simulink model "PMSM_PLL_MTPA"  (R2018b)
settings: Solver=VariableStepAuto  StartTime=0.0  StopTime=20  FixedStep=Ts  RelTol=1e-4  EnableMultiTasking=on
InitFcn:
  | Ts = 1e-4;
  | 
  | Rs = 0.8975;
  | Ld = 15e-3;
  | Lq = 19e-3;
  | Pn = 3;
  | flux = 0.1764;
  | 
  | Kp_PLL = 150;
  | Ki_PLL = 100;
undefined symbols (not defined in the file or in its folder): DiscIntNeverNeededParam
libraries: powerlib x5, powerlib_extras x2, simulink x2
settings Model: Creator=SUN  LastModifiedBy=liangjin
settings SolverCC: ZeroCrossControl=DisableAll
settings DataIOCC: LimitDataPoints=on  SaveFormat=Array
settings OptimizationCC: ExpressionDepthLimit=2147483647  InitFltsAndDblsToZero=on  LifeSpan=inf
settings DebuggingCC: UnderspecifiedInitializationDetection=Classic  MergeDetectMultiDrivingBlocksExec=none  SolverPrmCheckMsg=warning  FcnCallInpInsideContextMsg=warning  StateNameClashWarn=warning  SFUnexpectedBacktrackingDiag=warning  SFNoUnconditionalDefaultTransitionDiag=warning  SFExecutionAtInitializationDiag=none
settings HardwareCC: ProdBitPerPointer=32  ProdBitPerSizeT=32  ProdBitPerPtrDiffT=32  ProdLargestAtomicFloat=None  ProdIntDivRoundTo=Undefined  ProdEndianess=Unspecified  ProdWordSize=32  ProdHWDeviceType=32-bit Generic
settings ModelReferenceCC: PropagateSignalLabelsOutOfModel=off
settings SFSimCC: SimUseLocalCustomCode=off
settings RTWCC: RTWUseLocalCustomCode=off
settings CodeAppCC: StateflowObjectComments=on
settings GRTTargetCC: TargetLangStandard=C89/C90 (ANSI)  GeneratePreprocessorConditionals=Disable all  CombineOutputUpdateFcns=off  GRTInterface=on
settings ConfigComp: CovMetricSettings=dw  CovHtmlReporting=on  CovSaveCumulativeToWorkspaceVar=on  CovSaveSingleToWorkspaceVar=on  CovExternalEMLEnable=off  CovSFcnEnable=off
settings SimscapeCC: SimscapeNormalizeSystem=off

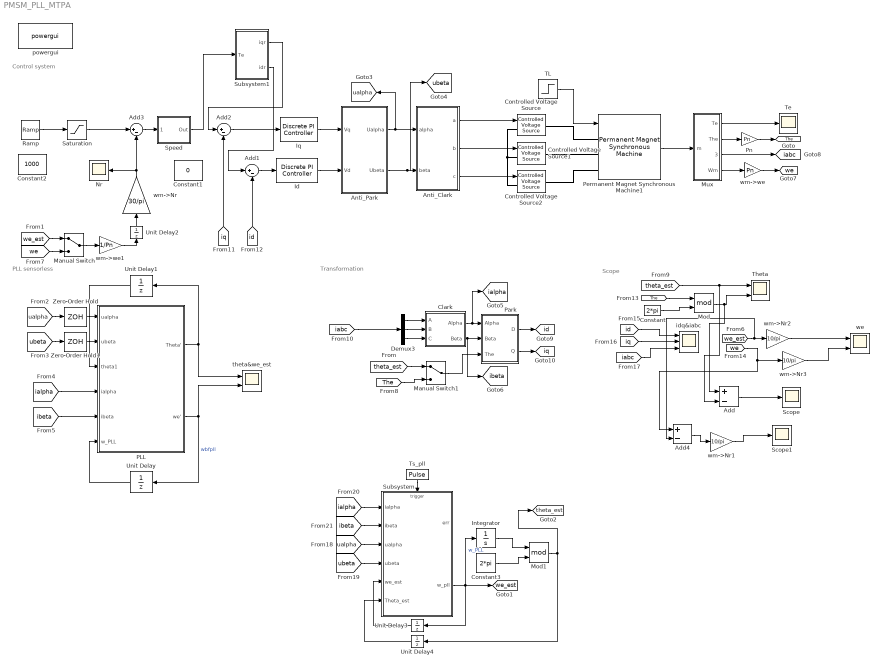
== system PMSM_PLL_MTPA ==
  note: Scope
  note: Control system
  note: Transformation
  note: PLL sensorless
  Add : Sum  Inputs=+-
  Add1 : Sum  Inputs=|+-
  Add2 : Sum  Inputs=|+-
  Add3 : Sum  Inputs=|+-
  Add4 : Sum  Inputs=+-
  Anti_Clark : Subsystem
  Anti_Park : Subsystem
  Clark : Subsystem
  Constant : Constant  Value=2*pi
  Constant1 : Constant  Value=0
  Constant2 : Constant  Value=1000
  Constant3 : Constant  Value=2*pi
  Controlled Voltage Source : powerlib/Electrical Sources/Controlled Voltage Source  Initialize=on  Source_Type=AC  Amplitude=0  Phase=0  Frequency=0  Measurements=None
      settings: SourceProductName=Simscape Electrical
  Controlled Voltage Source1 : powerlib/Electrical Sources/Controlled Voltage Source  Initialize=on  Source_Type=AC  Amplitude=0  Phase=0  Frequency=0  Measurements=None
      settings: SourceProductName=Simscape Electrical
  Controlled Voltage Source2 : powerlib/Electrical Sources/Controlled Voltage Source  Initialize=on  Source_Type=AC  Amplitude=0  Phase=0  Frequency=0  Measurements=None
      settings: SourceProductName=Simscape Electrical
  Demux3 : Demux  Outputs=3
  Id : powerlib_extras/Discrete  Control Blocks/Discrete PI Controller  Kp=Ld*376  Ki=Rs*376  Par_Limits=[311*0.9*sqrt(1/3) -311*0.9*sqrt(1/3)]  Init=0  Ts=Ts
  Integrator : Integrator
  Iq : powerlib_extras/Discrete  Control Blocks/Discrete PI Controller  Kp=Lq*376  Ki=Rs*376  Par_Limits=[311*0.9*sqrt(1/3) -311*0.9*sqrt(1/3)]  Init=0  Ts=Ts
  Manual Switch : ManualSwitch
  Manual Switch1 : ManualSwitch
  Mod : Math  Operator=mod  SaturateOnIntegerOverflow=on
  Mod1 : Math  Operator=mod  SaturateOnIntegerOverflow=on
  Mux : Subsystem
  Nr : Scope
  PLL : Subsystem
  Park : Subsystem
  Permanent Magnet Synchronous Machine1 : powerlib/Machines/Permanent Magnet Synchronous Machine  NbPhases=3  FluxDistribution=Sinusoidal  RotorType=Salient-pole  MechanicalLoad=Torque Tm  PresetModel=No  ShowDetailedParameters=on  MeasurementBus=off  Resistance=0.8975  Inductance=8.5e-3  dqInductances=[1.3*15e-3,1.3*19e-3]  La=0.000835  MachineConstant=Flux linkage established by magnets (V.s)  Flux=0.1764  VoltageCst=95.9863  TorqueCst=0.7938  Flat=120  Mechanical=[0.000311 0.0000001 3]  PolePairs=3  InitialConditions=[0,0, 0,0]  InitialConditions5ph=[0 0 0 0 0 0]  TsPowergui=0  TsBlock=Ts  RefAngle=Aligned with phase A axis (original Park)
  Pn : Gain  Gain=Pn
  Ramp : simulink/Sources/Ramp  slope=250  start=0  InitialOutput=0
  Saturation : Saturate  UpperLimit=1000  LowerLimit=-1000
  Scope : Scope
  Scope1 : Scope
  Speed : Subsystem  AncestorBlock=|  DialogController=POWERSYS.PowerSysDialog  mask(Discrete PI Controller){Kpw=0.01, Kiw=0.01*50, Ba=0, Par_Limits=[30 -30], Init=0, Ts=Ts*10}
      | powerlib_extras/Discrete 
      | Control Blocks/Discrete
      | PI Controller
      mask prompts: Kpw "Proportional gain (Kp):"; Kiw "Integral gain (Ki):"; Ba "feedback gain (Ba)"; Par_Limits "Output limits: [ Upper   Lower ]"; Init "Output initial value:"; Ts "Sample time:"
      mask help: This block implements a discrete PI controller.
      mask init:
      | UpperLimit=Par_Limits(1);
      | LowerLimit=Par_Limits(2);
      | power_initmask();
      mask Help: This block is part of a subset of blocks in the Extras library that does not have documentation associated with it, other than the block mask description.
      mask Display: disp('PI');
  Subsystem : Subsystem
  Subsystem1 : Subsystem
  TL : Step  Time=5  After=3  SampleTime=Ts
  Te : Scope
  Theta : Scope  NumInputPorts=2
  Ts_pll : DiscretePulseGenerator  PulseType=Time based  Period=Ts  PulseWidth=50
  Unit Delay{,1,3..4} (4 alike) : UnitDelay  SampleTime=Ts
  Unit Delay2 : UnitDelay  SampleTime=-1
  Zero-Order Hold : ZeroOrderHold  SampleTime=Ts
  Zero-Order Hold1 : ZeroOrderHold  SampleTime=Ts
  idq&iabc : Scope  NumInputPorts=3
  powergui : powerlib/powergui  SimulationMode=Continuous  SampleTime=Ts*10  frequency=60  Iterations=50  frequencyindice=0  Pbase=100e6  ErrMax=1e-4  UnitsV=kV  UnitsW=MW  buscounter=0  FunctionMessages=off  echomessages=off  EnableUseOfTLC=off  CurrentSourceSwitches=off  DisableSnubberDevices=off  DisableRonSwitches=off  DisableVfSwitches=off  DisplayEquations=off  SolverType=Tustin/Backward Euler (TBE)  Interpol=off  ExternalGateDelay=off  methode=off  Ts=100  x0status=blocks  SPID=off  SwTol=0  HookPort=off  RestoreLinks=warning  ResistiveCurrentMeasurement=off  Frange=[0:2:500]  Ylog=off  Xlog=on  ShowGrid=off  save=off  variable=ZData  structure=0  ZoomFFT=on  StartTime=0.0  cycles=1  DisplayStyle=1  fundamental=60  FreqAxis=off  MaxFrequency=1000  frequencyindicesteady=1  RmsSteady=1  display=off
  theta&we_est : Scope  NumInputPorts=2
  we : Scope  NumInputPorts=2
  wm->Nr : Gain  Gain=30/pi
  wm->Nr1 : Gain  Gain=10/pi
  wm->Nr2 : Gain  Gain=10/pi
  wm->Nr3 : Gain  Gain=10/pi
  wm->we : Gain  Gain=Pn
  wm->we1 : Gain  Gain=1/Pn
  tag scope: The=global, iabc=global, ialpha=global, ibeta=global, id=global, iq=global, theta_est=global, ualpha=global, ubeta=global, we=global, we_est=global
  wires:
  TL/1 -> Permanent Magnet Synchronous Machine1/1
  Permanent Magnet Synchronous Machine1/1 -> Mux/1(m)
  Add3/1 -> Speed/1(Error)
  Add1/1 -> Id/1
  wm->Nr/1 -> Add3/2, Nr/1
  Add2/1 -> Iq/1
  Mux/1(Te) -> Te/1
  Mux/2(The) -> Pn/1
  Pn/1 -> [The]
  Mux/4(Wm) -> wm->we/1
  Mux/3(Iabc) -> [iabc]
  Clark/1(Alpha) -> [ialpha], Park/1(Alpha)
  Demux3/1 -> Clark/1(A)
  Demux3/2 -> Clark/2(B)
  Demux3/3 -> Clark/3(C)
  Clark/2(Beta) -> Park/2(Beta), [ibeta]
  Iq/1 -> Anti_Park/1(Vq)
  Id/1 -> Anti_Park/2(Vd)
  Anti_Clark/1(a) -> Controlled Voltage Source/1
  Anti_Clark/2(b) -> Controlled Voltage Source1/1
  Anti_Clark/3(c) -> Controlled Voltage Source2/1
  PLL/2(we') -> Unit Delay/1, theta&we_est/2  "wbfpll"
  PLL/1(Theta') -> theta&we_est/1, Unit Delay1/1
  Constant/1 -> Mod/2
  Mod/1 -> Add/1, Theta/2
  Unit Delay/1 -> PLL/6(w_PLL)
  Unit Delay1/1 -> PLL/3(theta1)
  wm->we/1 -> [we]
  Ramp/1 -> Saturation/1
  [ialpha] -> PLL/4(ialpha)
  [ibeta] -> PLL/5(ibeta)
  Anti_Park/1(Ualpha) -> [ualpha], Anti_Clark/1(alpha)
  Anti_Park/2(Ubeta) -> [ubeta], Anti_Clark/2(beta)
  [we_est] -> Manual Switch/1
  [we] -> Manual Switch/2
  [theta_est] -> Manual Switch1/1
  Manual Switch1/1 -> Park/3(The)
  [The] -> Manual Switch1/2
  [ualpha] -> Zero-Order Hold/1
  Zero-Order Hold/1 -> PLL/1(ualpha)
  [ubeta] -> Zero-Order Hold1/1
  Zero-Order Hold1/1 -> PLL/2(ubeta)
  [theta_est] -> Add/2, Theta/1
  [iabc] -> Demux3/1
  Park/1(D) -> [id]
  Park/2(Q) -> [iq]
  [The] -> Mod/1
  [id] -> idq&iabc/1
  [iq] -> idq&iabc/2
  [iabc] -> idq&iabc/3
  [id] -> Add1/2
  [iq] -> Add2/2
  Manual Switch/1 -> wm->we1/1
  Add4/1 -> wm->Nr1/1
  wm->Nr1/1 -> Scope1/1
  [we] -> Add4/1, wm->Nr3/1
  [we_est] -> Add4/2, wm->Nr2/1
  Add/1 -> Scope/1
  wm->Nr2/1 -> we/1
  wm->Nr3/1 -> we/2
  wm->we1/1 -> Unit Delay2/1
  Unit Delay2/1 -> wm->Nr/1
  Saturation/1 -> Add3/1
  [ialpha] -> Subsystem/1(ialpha)
  [ibeta] -> Subsystem/2(ibeta)
  [ualpha] -> Subsystem/3(ualpha)
  [ubeta] -> Subsystem/4(ubeta)
  Ts_pll/1 -> Subsystem/Trigger
  Constant3/1 -> Mod1/2
  Integrator/1 -> Mod1/1
  Subsystem/2(w_pll) -> [we_est], Integrator/1, Unit Delay3/1  "w_PLL"
  Mod1/1 -> Unit Delay4/1, [theta_est]
  Unit Delay3/1 -> Subsystem/5(we_est)
  Unit Delay4/1 -> Subsystem/6(Theta_est)
  Speed/1(Out) -> Subsystem1/1(Te)
  Subsystem1/1(iqr) -> Add2/1
  Subsystem1/2(idr) -> Add1/1
  connections:
  Controlled Voltage Source/LConn1 -- Controlled Voltage Source2/LConn1 -- Controlled Voltage Source1/LConn1
  Controlled Voltage Source/RConn1 -- Permanent Magnet Synchronous Machine1/LConn1
  Controlled Voltage Source1/RConn1 -- Permanent Magnet Synchronous Machine1/LConn2
  Controlled Voltage Source2/RConn1 -- Permanent Magnet Synchronous Machine1/LConn3

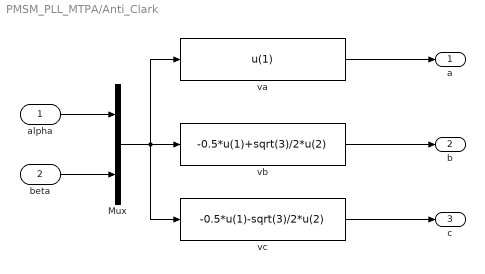
== system PMSM_PLL_MTPA/Anti_Clark ==
  alpha : Inport
  beta : Inport  Port=2
  Mux : Mux  Inputs=2
  va : Fcn  Expr=u(1)
  vb : Fcn  Expr=-0.5*u(1)+sqrt(3)/2*u(2)
  vc : Fcn  Expr=-0.5*u(1)-sqrt(3)/2*u(2)
  a : Outport
  b : Outport  Port=2
  c : Outport  Port=3
  wires:
  va/1 -> a/1
  beta/1 -> Mux/2
  alpha/1 -> Mux/1
  Mux/1 -> vc/1, vb/1, va/1
  vb/1 -> b/1
  vc/1 -> c/1

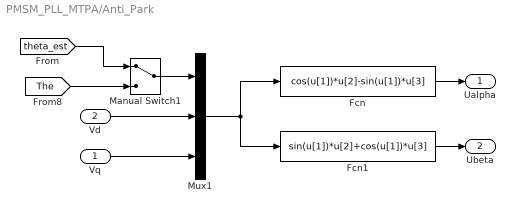
== system PMSM_PLL_MTPA/Anti_Park ==
  Vq : Inport
  Vd : Inport  Port=2
  Fcn : Fcn  Expr=cos(u[1])*u[2]-sin(u[1])*u[3]
  Fcn1 : Fcn  Expr=sin(u[1])*u[2]+cos(u[1])*u[3]
  Manual Switch1 : ManualSwitch
  Mux1 : Mux  Inputs=3
  Ualpha : Outport
  Ubeta : Outport  Port=2
  wires:
  Fcn1/1 -> Ubeta/1
  Fcn/1 -> Ualpha/1
  Mux1/1 -> Fcn/1, Fcn1/1
  Vd/1 -> Mux1/2
  Vq/1 -> Mux1/3
  Manual Switch1/1 -> Mux1/1
  [The] -> Manual Switch1/2
  [theta_est] -> Manual Switch1/1

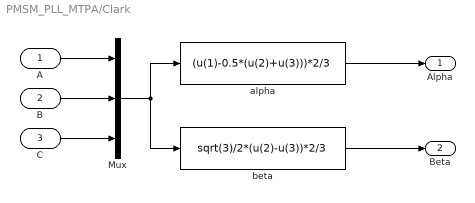
== system PMSM_PLL_MTPA/Clark ==
  A : Inport
  B : Inport  Port=2
  C : Inport  Port=3
  Mux : Mux  Inputs=3
  alpha : Fcn  Expr=(u(1)-0.5*(u(2)+u(3)))*2/3
  beta : Fcn  Expr=sqrt(3)/2*(u(2)-u(3))*2/3
  Alpha : Outport
  Beta : Outport  Port=2
  wires:
  alpha/1 -> Alpha/1
  B/1 -> Mux/2
  C/1 -> Mux/3
  A/1 -> Mux/1
  Mux/1 -> beta/1, alpha/1
  beta/1 -> Beta/1

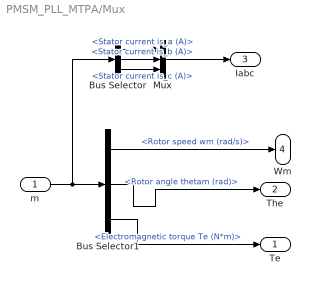
== system PMSM_PLL_MTPA/Mux ==
  m : Inport
  Bus Selector : BusSelector  OutputSignals=Stator current is_a (A),Stator current is_b (A),Stator current is_c (A)
  Bus Selector1 : BusSelector  OutputSignals=Rotor speed wm (rad/s),Rotor angle thetam (rad),Electromagnetic torque Te (N*m)
  Mux : Mux  Inputs=3
  Te : Outport
  The : Outport  Port=2
  Iabc : Outport  Port=3
  Wm : Outport  Port=4
  wires:
  Bus Selector1/1 -> Wm/1  "<Rotor speed wm (rad/s)>"
  Bus Selector1/2 -> The/1  "<Rotor angle thetam (rad)>"
  Bus Selector1/3 -> Te/1  "<Electromagnetic torque Te (N*m)>"
  m/1 -> Bus Selector/1, Bus Selector1/1
  Bus Selector/2 -> Mux/2  "<Stator current is_b (A)>"
  Bus Selector/3 -> Mux/3  "<Stator current is_c (A)>"
  Bus Selector/1 -> Mux/1  "<Stator current is_a (A)>"
  Mux/1 -> Iabc/1

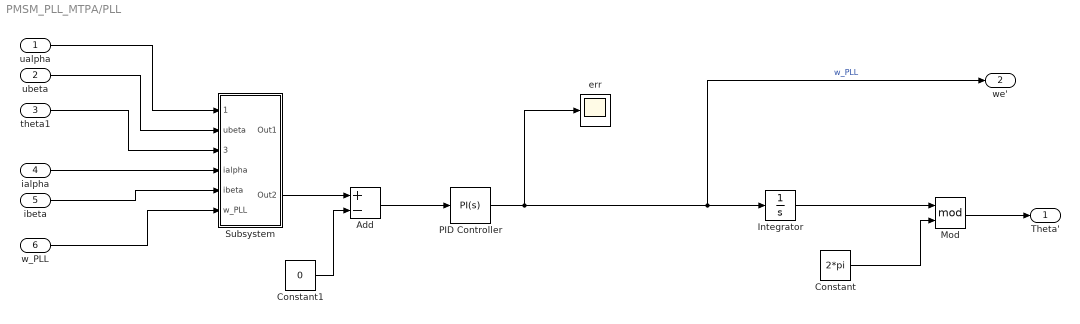
== system PMSM_PLL_MTPA/PLL ==
  ualpha : Inport
  ubeta : Inport  Port=2
  theta1 : Inport  Port=3
  ialpha : Inport  Port=4
  ibeta : Inport  Port=5
  w_PLL : Inport  Port=6
  Add : Sum  Inputs=+-
  Constant : Constant  Value=2*pi
  Constant1 : Constant  Value=0
  Integrator : Integrator
  Mod : Math  Operator=mod  SaturateOnIntegerOverflow=on
  PID Controller : simulink/Continuous/PID Controller  Controller=PI  Form=Parallel  TimeDomain=Continuous-time  SampleTime=-1  IntegratorMethod=Forward Euler  FilterMethod=Forward Euler  ControllerParametersSource=internal  P=Kp_PLL  I=Ki_PLL  D=0  UseFilter=on  N=100  TunerSelectOption=Transfer Function Based (PID Tuner App)  InitialConditionSource=internal  InitialConditionForIntegrator=0  InitialConditionForFilter=0  DifferentiatorICPrevScaledInput=0  ExternalReset=none  TrackingMode=off  Kt=1  LimitOutput=off  UpperSaturationLimit=inf  LowerSaturationLimit=-inf  LinearizeAsGain=on  AntiWindupMode=none  Kb=1  POutMin=[]  POutMax=[]  IOutMin=[]  IOutMax=[]  DOutMin=[]  DOutMax=[]  NOutMin=[]  NOutMax=[]  SumOutMin=[]  SumOutMax=[]  SaturationOutMin=[]  SaturationOutMax=[]  PParamMin=[]  PParamMax=[]  IParamMin=[]  IParamMax=[]  DParamMin=[]  DParamMax=[]  NParamMin=[]  NParamMax=[]  KbParamMin=[]  KbParamMax=[]  KtParamMin=[]  KtParamMax=[]  KbOutMin=[]  KbOutMax=[]  KtOutMin=[]  KtOutMax=[]  IntegratorOutMin=[]  IntegratorOutMax=[]  FilterOutMin=[]  FilterOutMax=[]  SumI1OutMin=[]  SumI1OutMax=[]  SumI2OutMin=[]  SumI2OutMax=[]  SumI3OutMin=[]  SumI3OutMax=[]  SumI4OutMin=[]  SumI4OutMax=[]  SumDOutMin=[]  SumDOutMax=[]  DifferentiatorOutMin=[]  DifferentiatorOutMax=[]  FilterDiffOutCoefMin=[]  FilterDiffOutCoefMax=[]  ReciprocalOutMin=[]  ReciprocalOutMax=[]  SumDenOutMin=[]  SumDenOutMax=[]  SumNumOutMin=[]  SumNumOutMax=[]  DivideOutMin=[]  DivideOutMax=[]  IntegratorContinuousStateAttributes=''  IntegratorStateMustResolveToSignalObject=off  IntegratorRTWStateStorageClass=Auto  FilterContinuousStateAttributes=''  FilterStateMustResolveToSignalObject=off  FilterRTWStateStorageClass=Auto  ParallelPVariant=InternalParameters  IdealPVariant=Disabled  IVariant=InternalParameters  DVariant=Disabled  IntegratorVariant=Continuous  SatVariant=Disabled  AWVariant=Passthrough  PCopyVariant=Disabled  TRVariant=Disabled  FdbkBlocksVariant=Forward  IdealPFdbkVariant=Disabled  SatFdbkVariant=Disabled  DerivativeFilterVariant=Disabled  NVariant=Disabled  NCopyVariant=Disabled_SignalSpec  FilterICVariant=Disabled  IntegratorICVariant=InternalICs  ExternalResetVariant=Disabled  TRSumVariant=Passthrough  SumFdbkVariant=Disabled  SumVariant=Sum_PI
  Subsystem : Subsystem
  err : Scope
  Theta' : Outport
  we' : Outport  Port=2
  wires:
  Constant/1 -> Mod/2
  Integrator/1 -> Mod/1
  Mod/1 -> Theta'/1
  ualpha/1 -> Subsystem/1(ualpha)
  ubeta/1 -> Subsystem/2(ubeta)
  ialpha/1 -> Subsystem/4(ialpha)
  ibeta/1 -> Subsystem/5(ibeta)
  theta1/1 -> Subsystem/3(theta1)
  w_PLL/1 -> Subsystem/6(w_PLL)
  Subsystem/2(Out2) -> Add/1
  Constant1/1 -> Add/2
  Add/1 -> PID Controller/1
  PID Controller/1 -> we'/1, Integrator/1, err/1  "w_PLL"

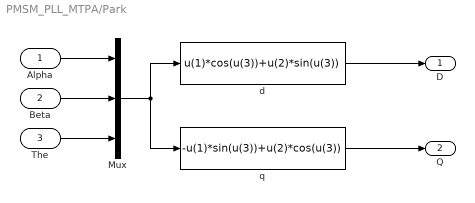
== system PMSM_PLL_MTPA/Park ==
  Alpha : Inport
  Beta : Inport  Port=2
  The : Inport  Port=3
  Mux : Mux  Inputs=3
  d : Fcn  Expr=u(1)*cos(u(3))+u(2)*sin(u(3))
  q : Fcn  Expr=-u(1)*sin(u(3))+u(2)*cos(u(3))
  D : Outport
  Q : Outport  Port=2
  wires:
  d/1 -> D/1
  Beta/1 -> Mux/2
  Alpha/1 -> Mux/1
  Mux/1 -> q/1, d/1
  q/1 -> Q/1
  The/1 -> Mux/3

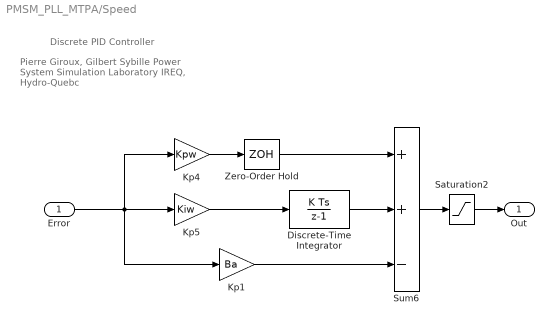
== system PMSM_PLL_MTPA/Speed ==
  note: Discrete PID Controller
  note: Pierre Giroux, Gilbert Sybille
      | Power System Simulation Laboratory
      | IREQ, Hydro-Quebc
  Error : Inport  SampleTime=Ts
  Discrete-Time Integrator : DiscreteIntegrator  InitialCondition=Init  SampleTime=Ts  LimitOutput=on  UpperSaturationLimit=UpperLimit  LowerSaturationLimit=LowerLimit  ICPrevOutput=DiscIntNeverNeededParam  ICPrevScaledInput=DiscIntNeverNeededParam
  Kp1 : Gain  Gain=Ba  SampleTime=Ts  SaturateOnIntegerOverflow=on  OutDataTypeStr=Inherit: Same as input  ParamDataTypeStr=Inherit: Same as input
  Kp4 : Gain  Gain=Kpw  SampleTime=Ts  SaturateOnIntegerOverflow=on  OutDataTypeStr=Inherit: Same as input  ParamDataTypeStr=Inherit: Same as input
  Kp5 : Gain  Gain=Kiw  SampleTime=Ts  SaturateOnIntegerOverflow=on  OutDataTypeStr=Inherit: Same as input  ParamDataTypeStr=Inherit: Same as input
  Saturation2 : Saturate  UpperLimit=UpperLimit  LowerLimit=LowerLimit  SampleTime=Ts
  Sum6 : Sum  Inputs=++-  SampleTime=Ts  SaturateOnIntegerOverflow=on  InputSameDT=on  OutDataTypeStr=Inherit: Same as first input
  Zero-Order Hold : ZeroOrderHold  SampleTime=Ts
  Out : Outport  SampleTime=Ts  InitialOutput=0
  wires:
  Error/1 -> Kp1/1, Kp5/1, Kp4/1
  Zero-Order Hold/1 -> Sum6/1
  Saturation2/1 -> Out/1
  Discrete-Time Integrator/1 -> Sum6/2
  Kp4/1 -> Zero-Order Hold/1
  Kp5/1 -> Discrete-Time Integrator/1
  Sum6/1 -> Saturation2/1
  Kp1/1 -> Sum6/3

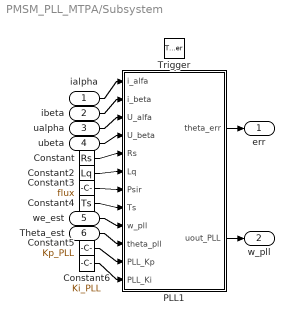
== system PMSM_PLL_MTPA/Subsystem ==
  ialpha : Inport
  ibeta : Inport  Port=2
  ualpha : Inport  Port=3
  ubeta : Inport  Port=4
  we_est : Inport  Port=5
  Theta_est : Inport  Port=6
  Trigger : TriggerPort  VariantControl=Variant  PortDimensions=1
  Constant : Constant  Value=Rs
  Constant2 : Constant  Value=Lq
  Constant3 : Constant  Value=flux
  Constant4 : Constant  Value=Ts
  Constant5 : Constant  Value=Kp_PLL
  Constant6 : Constant  Value=Ki_PLL
  PLL1 : MATLAB Function  TreatAsAtomicUnit=on
  err : Outport
  w_pll : Outport  Port=2
  wires:
  PLL1/1(theta_err) -> err/1
  ialpha/1 -> PLL1/1(i_alfa)
  we_est/1 -> PLL1/9(w_pll)
  Constant/1 -> PLL1/5(Rs)
  Constant2/1 -> PLL1/6(Lq)
  ualpha/1 -> PLL1/3(U_alfa)
  ibeta/1 -> PLL1/2(i_beta)
  ubeta/1 -> PLL1/4(U_beta)
  Constant3/1 -> PLL1/7(Psir)
  Theta_est/1 -> PLL1/10(theta_pll)
  Constant4/1 -> PLL1/8(Ts)
  Constant6/1 -> PLL1/12(PLL_Ki)
  Constant5/1 -> PLL1/11(PLL_Kp)
  PLL1/2(uout_PLL) -> w_pll/1

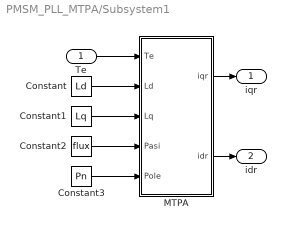
== system PMSM_PLL_MTPA/Subsystem1 ==
  Te : Inport
  Constant : Constant  Value=Ld
  Constant1 : Constant  Value=Lq
  Constant2 : Constant  Value=flux
  Constant3 : Constant  Value=Pn
  MTPA : MATLAB Function  TreatAsAtomicUnit=on
  iqr : Outport
  idr : Outport  Port=2
  wires:
  MTPA/2(idr) -> idr/1
  MTPA/1(iqr) -> iqr/1
  Te/1 -> MTPA/1(Te)
  Constant/1 -> MTPA/2(Ld)
  Constant1/1 -> MTPA/3(Lq)
  Constant3/1 -> MTPA/5(Pole)
  Constant2/1 -> MTPA/4(Pasi)

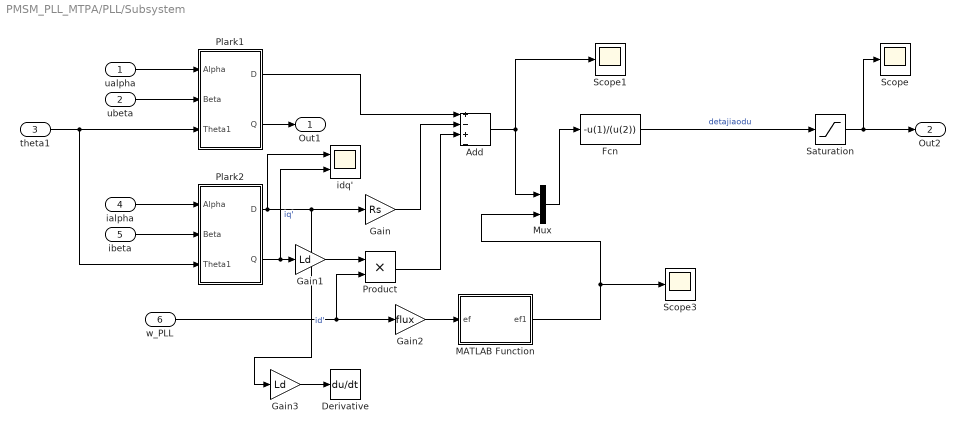
== system PMSM_PLL_MTPA/PLL/Subsystem ==
  ualpha : Inport
  ubeta : Inport  Port=2
  theta1 : Inport  Port=3
  ialpha : Inport  Port=4
  ibeta : Inport  Port=5
  w_PLL : Inport  Port=6
  Add : Sum  Inputs=+-+-
  Derivative : Derivative
  Fcn : Fcn  Expr=-u(1)/(u(2))
  Gain : Gain  Gain=Rs
  Gain1 : Gain  Gain=Ld
  Gain2 : Gain  Gain=flux
  Gain3 : Gain  Gain=Ld
  MATLAB Function : MATLAB Function  TreatAsAtomicUnit=on
  Mux : Mux  Inputs=2
  Plark1 : Subsystem
  Plark2 : Subsystem
  Product : Product
  Saturation : Saturate  UpperLimit=1  LowerLimit=-1
  Scope : Scope
  Scope1 : Scope
  Scope3 : Scope
  idq' : Scope  NumInputPorts=2
  Out1 : Outport
  Out2 : Outport  Port=2
  wires:
  Product/1 -> Add/3
  ubeta/1 -> Plark1/2(Beta)
  w_PLL/1 -> Gain2/1, Product/2
  theta1/1 -> Plark2/3(Theta1), Plark1/3(Theta1)
  Fcn/1 -> Saturation/1  "detajiaodu"
  Add/1 -> Scope1/1, Mux/1
  Mux/1 -> Fcn/1
  Gain/1 -> Add/2
  Plark1/1(D) -> Add/1
  Plark1/2(Q) -> Out1/1
  ialpha/1 -> Plark2/1(Alpha)
  Plark2/1(D) -> Gain/1, Gain3/1, idq'/1  "id'"
  Plark2/2(Q) -> idq'/2, Gain1/1  "iq'"
  ualpha/1 -> Plark1/1(Alpha)
  ibeta/1 -> Plark2/2(Beta)
  Gain1/1 -> Product/1
  Gain2/1 -> MATLAB Function/1(ef)
  Saturation/1 -> Out2/1, Scope/1
  MATLAB Function/1(ef1) -> Mux/2, Scope3/1
  Gain3/1 -> Derivative/1

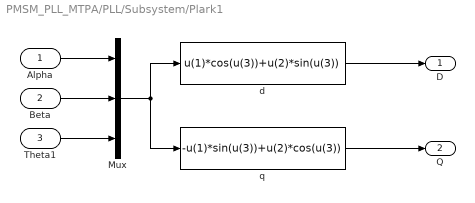
== system PMSM_PLL_MTPA/PLL/Subsystem/Plark1 ==
  Alpha : Inport
  Beta : Inport  Port=2
  Theta1 : Inport  Port=3
  Mux : Mux  Inputs=3
  d : Fcn  Expr=u(1)*cos(u(3))+u(2)*sin(u(3))
  q : Fcn  Expr=-u(1)*sin(u(3))+u(2)*cos(u(3))
  D : Outport
  Q : Outport  Port=2
  wires:
  d/1 -> D/1
  Beta/1 -> Mux/2
  Alpha/1 -> Mux/1
  Mux/1 -> q/1, d/1
  q/1 -> Q/1
  Theta1/1 -> Mux/3

== system PMSM_PLL_MTPA/PLL/Subsystem/Plark2 ==
  Alpha : Inport
  Beta : Inport  Port=2
  Theta1 : Inport  Port=3
  Mux : Mux  Inputs=3
  d : Fcn  Expr=u(1)*cos(u(3))+u(2)*sin(u(3))
  q : Fcn  Expr=-u(1)*sin(u(3))+u(2)*cos(u(3))
  D : Outport
  Q : Outport  Port=2
  wires:
  Theta1/1 -> Mux/3
  q/1 -> Q/1
  Mux/1 -> d/1, q/1
  Alpha/1 -> Mux/1
  Beta/1 -> Mux/2
  d/1 -> D/1

== matlab function PMSM_PLL_MTPA/Subsystem1/MTPA ==
  data: iqr output; Te input; idr output; Ld input; Lq input; Pasi input; Pole input
function [iqr,idr] = MTPA(Te,Ld,Lq,Pasi,Pole)

persistent id1 iq1 temp1 temp2 temp3;

if isempty(id1)
    id1=0;iq1=0;temp1=0;temp2=0;temp3 = 0;
end
temp1 = Pasi.^2 - 4*(Ld-Lq).^2;
temp2 = 8*Te*Pasi/(3*Pole);
temp3 = temp2.^2-4*temp1*((4*Te/3/Pole).^2-Pasi.^2);

if (temp3 < 0)
    temp3 = 0;
end

iq1 = (temp2 + sqrt(temp3))/(2*temp1);
id1 = Pasi/(2*Lq-2*Ld) - sqrt((Pasi/(2*Lq-2*Ld)).^2+iq1.^2);

if (id1<-30)
    id1 = -30;
elseif (id1>30)
    id1 = 30;
end

if (iq1<-30)
    iq1 = -30;
elseif (iq1>30)
    iq1 = 30;
end
idr = id1;
iqr = iq1;

== matlab function PMSM_PLL_MTPA/PLL/Subsystem/MATLAB Function ==
  data: ef input; ef1 output
function ef1 = sat_(ef)
if ((ef>=0) && (ef<10))
    ef = 10;
elseif ((ef<0) && (ef>(-10)))
    ef = -10;
end
ef1 = ef;

== matlab function PMSM_PLL_MTPA/Subsystem/PLL1 ==
  data: theta_err output; i_alfa input; i_beta input; U_alfa input; U_beta input; Rs input; uout_PLL output; Lq input; Psir input; Ts input; w_pll input; theta_pll input; PLL_Kp input; PLL_Ki input
function [theta_err, uout_PLL]      = PLL(i_alfa,i_beta,U_alfa,U_beta,Rs,Lq,Psir,Ts,w_pll,theta_pll,PLL_Kp,PLL_Ki)


% refer 'Rolando' "Edsigh and Evaluation of PLL"
persistent id1 ui_PLL w_pll_f;
if isempty(id1)    
   id1=0;ui_PLL=0;w_pll_f=0;
end
% U_alfa/beta -> Ud/q ,i_alfa/beta -> id/q
x1=theta_pll;
Ud= cos(x1)*U_alfa+sin(x1)*U_beta;
Uq=-sin(x1)*U_alfa+cos(x1)*U_beta;
id= cos(x1)*i_alfa+sin(x1)*i_beta;
iq=-sin(x1)*i_alfa+cos(x1)*i_beta;

id2=id;
iq2=iq;

 w_pll_f =w_pll_f + 0.715*(w_pll-w_pll_f);

e_d=(Ud-Rs*id2+w_pll_f*Lq*iq2);
e_mod=(Psir)*w_pll_f;


if (e_mod>-10 && e_mod<0)
    e_mod =-10;
elseif (e_mod>=0 && e_mod<10)
    e_mod=10;
end


sin_=e_d/e_mod;

if sin_>1
    sin_=1;
elseif sin_<-1
    sin_=-1;
end


theta_err = -sin_;


out_d = -sin_;

%save for next
id1=id;
iq1=iq;

% PI  for PLL
ui_PLL = PLL_Ki *theta_err*Ts+ ui_PLL;
uout_PLL = PLL_Kp*theta_err + ui_PLL;

ui_PLL =uout_PLL - PLL_Kp*theta_err;
if uout_PLL == 0
    ui_PLL=0;
end
%ui_PLL = uout_PLL-PLL_Kp*err_pll;
